simulink model "task2"  (R2026a)
settings: Solver=FixedStepAuto  StopTime=6000  FixedStep=1
values from neighbouring files (symbols this model uses):
  a = 0.9    [modelParams.m]
  b = 0.98    [modelParams.m]
  k = -25    [modelParams.m]
  Ref = 180    [modelParams.m]
libraries: sl_discontinuities x1
settings Model: Creator=micha  LastModifiedBy=socks

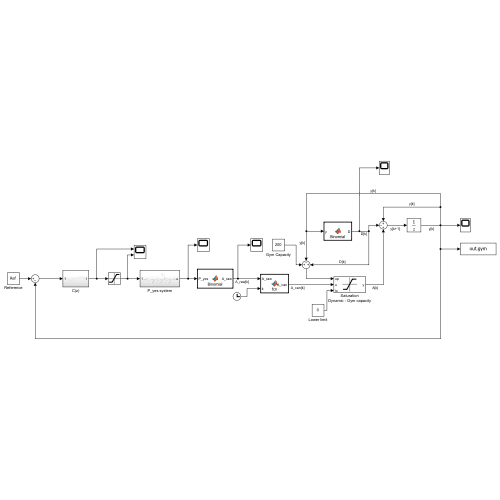
[thumbnail: Simulink's stored preview of the top-level diagram]
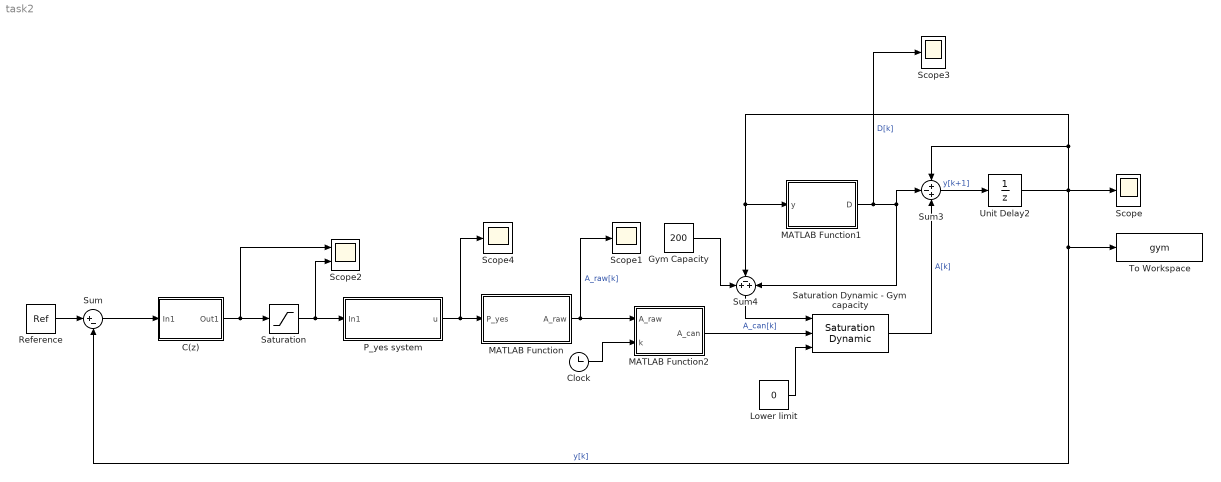
== system task2 ==
  C(z) : Subsystem
  Clock : Clock
  Gym Capacity : Constant  Value=200
  Lower limit : Constant  Value=0
  MATLAB Function : MATLAB Function  TreatAsAtomicUnit=on
  MATLAB Function1 : MATLAB Function  TreatAsAtomicUnit=on
  MATLAB Function2 : MATLAB Function  TreatAsAtomicUnit=on
  P_yes system : Subsystem
  Reference : Constant  Value=Ref
  Saturation : Saturate  UpperLimit=inf()  LowerLimit=0
  Saturation Dynamic - Gym capacity : sl_discontinuities/Saturation Dynamic  OutMin=[]  OutMax=[]  OutDataTypeStr=Inherit: Same as second input  OutDataType=fixdt(1, 16)  OutScaling=2^-10  DoSatur=off
  Scope{,1,3..4} (4 alike) : Scope
      Scope settings: ActiveDisplayYMinimum=-47.479792271127423  ActiveDisplayYMaximum=311.47685257771468
      Scope1 settings: ActiveDisplayYMinimum=14.339302507173556  ActiveDisplayYMaximum=22.469506034497716  DataLoggingVariableName=ScopeData2
      Scope3 settings: ActiveDisplayYMinimum=-50.4331308433664  ActiveDisplayYMaximum=130.86436698457749  DataLoggingVariableName=ScopeData3
      Scope4 settings: ActiveDisplayYMinimum=0.77614866296565965  ActiveDisplayYMaximum=0.99472795907058786  DataLoggingVariableName=ScopeData4
  Scope2 : Scope  NumInputPorts=2
      settings: ActiveDisplayYMinimum=-950.37565203468239  ActiveDisplayYMaximum=1900.3930464688765
  Sum : Sum  Inputs=|+-
  Sum3 : Sum  Inputs=+-+
  Sum4 : Sum  Inputs=+-+
  To Workspace : ToWorkspace  VariableName=gym  SaveFormat=Timeseries  SampleTime=-1
  Unit Delay2 : UnitDelay  SampleTime=-1
  wires:
  Reference/1 -> Sum/1
  P_yes system/1(u) -> Scope4/1, MATLAB Function/1(P_yes)
  Lower limit/1 -> Saturation Dynamic - Gym capacity/3
  Saturation Dynamic - Gym capacity/1 -> Sum3/3  "A[k]"
  Sum3/1 -> Unit Delay2/1  "y[k+1]"
  Unit Delay2/1 -> To Workspace/1, Sum/2, Scope/1, Sum4/2, MATLAB Function1/1(y), Sum3/1  "y[k]"
  MATLAB Function1/1(D) -> Scope3/1, Sum4/3, Sum3/2  "D[k]"
  Gym Capacity/1 -> Sum4/1
  Sum4/1 -> Saturation Dynamic - Gym capacity/1
  Sum/1 -> C(z)/1(In1)
  C(z)/1(Out1) -> Scope2/1, Saturation/1
  Saturation/1 -> P_yes system/1(In1), Scope2/2
  Clock/1 -> MATLAB Function2/2(k)
  MATLAB Function/1(A_raw) -> Scope1/1, MATLAB Function2/1(A_raw)  "A_raw[k]"
  MATLAB Function2/1(A_can) -> Saturation Dynamic - Gym capacity/2  "A_can[k]"

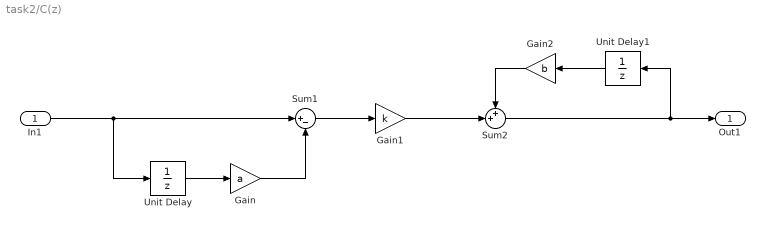
== system task2/C(z) ==
  In1 : Inport
  Gain : Gain  Gain=a
  Gain1 : Gain  Gain=k
  Gain2 : Gain  Gain=b
  Sum1 : Sum  Inputs=|+-
  Sum2 : Sum  Inputs=++|
  Unit Delay : UnitDelay  SampleTime=-1
  Unit Delay1 : UnitDelay  SampleTime=-1
  Out1 : Outport
  wires:
  Gain1/1 -> Sum2/2
  Gain2/1 -> Sum2/1
  Gain/1 -> Sum1/2
  Unit Delay/1 -> Gain/1
  Sum1/1 -> Gain1/1
  Unit Delay1/1 -> Gain2/1
  In1/1 -> Sum1/1, Unit Delay/1
  Sum2/1 -> Out1/1, Unit Delay1/1

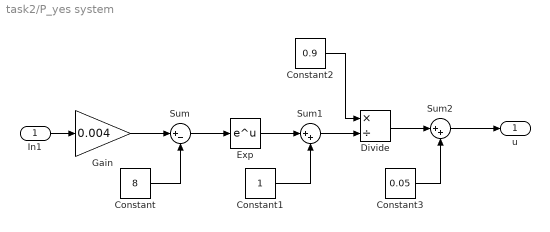
== system task2/P_yes system ==
  In1 : Inport
  Constant : Constant  Value=8
  Constant1 : Constant
  Constant2 : Constant  Value=0.9
  Constant3 : Constant  Value=0.05
  Divide : Product  Inputs=*/
  Exp : Math
  Gain : Gain  Gain=0.004
  Sum : Sum  Inputs=|+-
  Sum1 : Sum  Inputs=|++
  Sum2 : Sum  Inputs=|++
  u : Outport
  wires:
  In1/1 -> Gain/1
  Constant1/1 -> Sum1/2
  Exp/1 -> Sum1/1
  Sum/1 -> Exp/1
  Constant/1 -> Sum/2
  Gain/1 -> Sum/1
  Sum1/1 -> Divide/2
  Constant2/1 -> Divide/1
  Divide/1 -> Sum2/1
  Sum2/1 -> u/1
  Constant3/1 -> Sum2/2

== matlab function task2/MATLAB Function ==
  data: P_yes input; A_raw output
function A_raw = Binomial(P_yes)
    n = 20;
    trials = rand(1, n) < P_yes;
    A_raw = sum(trials);

end

== matlab function task2/MATLAB Function2 ==
  data: A_raw input; A_can output; k input
function A_can = fcn(A_raw, k)

    k_week = mod(k, 2016);

    if k_week < 1236
        open = 1;
    else 
        open = 0;
    end

    A_can = open * A_raw;

== matlab function task2/MATLAB Function1 ==
  data: y input; D output
function D = Binomial(y)
    trials = rand(1, y) < 0.1;
    D = sum(trials);
end
